simulink model "RRmanipulatorsim_"  (R2020a)
settings: Solver=VariableStepAuto  StartTime=0.0  StopTime=7  RelTol=1e-3
values from neighbouring files (symbols this model uses):
  ike = ke^(-1)    (= 1e-06)    [RRmanipulator.m]    (also in RRmanipulator_.m)
  Ke = [1e6 0; 0 0]    [RRmanipulator.m]    (also in RRmanipulator_.m)
  ke = 1e6    (= 1000000)    [RRmanipulator.m]    (also in RRmanipulator_.m)
  Kp = [g1 0; 0 g2]    [RRmanipulator.m]    (also in RRmanipulator_.m)
  Kpf = [g1f 0; 0 g2f]    [RRmanipulator.m]    (also in RRmanipulator_.m)
  Kpf_ = g1f    (= 500000)    [RRmanipulator.m]    (also in RRmanipulator_.m)
  Kv = [2*sqrt(g1) 0; 0 2*sqrt(g2)]    [RRmanipulator.m]    (also in RRmanipulator_.m)
  Kvf = [2*sqrt(g1f) 0; 0 2*sqrt(g2f)]    [RRmanipulator.m]    (also in RRmanipulator_.m)
  R = [cos(-pi/4) -sin(-pi/4) ... (first row only)    [RRmanipulator.m]    (also in RRmanipulator_.m)
  RT = R'    [RRmanipulator.m]    (also in RRmanipulator_.m)
  S = [0 0; 0 1]    [RRmanipulator.m]    (also in RRmanipulator_.m)
  S_ = [1 0; 0 0]    [RRmanipulator.m]    (also in RRmanipulator_.m)
libraries: roblocks x52, simulink x18
(part 2 of 3)

== matlab function RRmanipulatorsim_/MATLAB Function35 ==
  data: q input; taux output; qd input
function taux = Vx_Fx(q, qd)
    L = [1 1]; %Links long.
    m = [1 1]; %Links weight.
    
    M = [L(2)*m(2)*(L(2)+cos(q(2))*L(1))+m(1)*L(1)^2+L(1)*m(2)*(L(1)+cos(q(2))*L(2)) L(2)^2*m(2)+L(1)*m(2)*L(2)*cos(q(2));
        L(2)*m(2)*(L(2)+cos(q(2))*L(1)) L(2)^2*m(2)];
    V = [-2*m(2)*L(1)*L(2)*sin(q(2))*prod(qd)-m(2)*L(1)*L(2)*sin(q(2))*qd(2)^2;
        m(2)*L(1)*L(2)*sin(q(2))*qd(1)^2];
    G = [0;
        0];
    F = [sign(qd(1));
        sign(qd(2))];
    J = [-sin(sum(q))*L(2)-sin(q(1))*L(1) -sin(sum(q))*L(2);
        cos(sum(q))*L(2)+cos(q(1))*L(1) cos(sum(q))*L(2)];
    iJ = J^(-1);
    iJT = (J')^(-1);
    dJ = [-(sum(qd))*cos(sum(q))*L(2)-qd(1)*cos(q(1))*L(1) -(sum(qd))*cos(sum(q))*L(2);
        -(sum(qd))*sin(sum(q))*L(2)-qd(1)*sin(q(1))*L(1) -(sum(qd))*sin(sum(q))*L(2)];
    
    %dJqd = [dJ(1,1)*qd(1)+dJ(1,2)*qd(2); dJ(2,1)*qd(1)+dJ(2,2)*qd(2)];
    Vx = M*iJ*dJ;
    Vx = V - [Vx(1,1)*qd(1)+Vx(1,2)*qd(2); Vx(2,1)*qd(1)+Vx(2,2)*qd(2)];
    Vx = [iJT(1,1)*Vx(1)+iJT(1,2)*Vx(2); iJT(2,1)*Vx(1)+iJT(2,2)*Vx(2)];
    Gx = [iJT(1,1)*G(1)+iJT(1,2)*G(2); iJT(2,1)*G(1)+iJT(2,2)*G(2)];
    Fx = [iJT(1,1)*F(1)+iJT(1,2)*F(2); iJT(2,1)*F(1)+iJT(2,2)*F(2)];
taux = Vx + Gx + Fx;

% function taux = Vx_Fx(q, qd)
%     C = RRbot.coriolis(q', qd');
%     V = [C(1,1)*qd(1)+C(1,2)*qd(2); C(2,1)*qd(1)+C(2,2)*qd(2)]; %V = Cqd
%     F = -RRbot.friction(qd')';
%     J = RRbot.jacob0(q');
%     J = J(1:N,1:N);
%     iJ = J^(-1);
%     iJT = J.'^(-1);
%     dJ = [-(sum(qd))*cos(sum(q))*LT-qd(1)*cos(q(1))*L1 -(sum(qd))*cos(sum(q))*LT;
%         -(sum(qd))*sin(sum(q))*LT-qd(1)*sin(q(1))*L1 -(sum(qd))*sin(sum(q))*LT];
%     dJqd = [dJ(1,1)*qd(1)+dJ(1,2)*qd(2); dJ(2,1)*qd(1)+dJ(2,2)*qd(2)];
%     
%     Vx = M*iJ;
%     Vx = V - [Vx(1,1)*dJqd(1)+Vx(1,2)*dJqd(2); Vx(2,1)*dJqd(1)+Vx(2,2)*dJqd(2)];
%     Vx = [iJT(1,1)*Vx(1)+iJT(1,2)*Vx(2); iJT(2,1)*Vx(1)+iJT(2,2)*Vx(2)];
%     Fx = [iJT(1,1)*F(1)+iJT(1,2)*F(2); iJT(2,1)*F(1)+iJT(2,2)*F(2)];
% taux = Vx + Fx;

== matlab function RRmanipulatorsim_/MATLAB Function36 ==
  data: q input; x output
function x = kine(q)
    L = [1 1]; %Links long.

x = [cos(sum(q))*L(2)+cos(q(1))*L(1); sin(sum(q))*L(2)+sin(q(1))*L(1)];

== matlab function RRmanipulatorsim_/MATLAB Function37 ==
  data: q input; xd output; qd input
function xd = J(q, qd)
    L = [1 1]; %Links long.

    J = [-sin(sum(q))*L(2)-sin(q(1))*L(1) -sin(sum(q))*L(2);
        cos(sum(q))*L(2)+cos(q(1))*L(1) cos(sum(q))*L(2)];
xd = [J(1,1)*qd(1)+J(1,2)*qd(2); J(2,1)*qd(1)+J(2,2)*qd(2)];

== matlab function RRmanipulatorsim_/MATLAB Function38 ==
  data: q input; tau output; f input
function tau = JT(q, f)    
    L = [1 1]; %Links long.

    J = [-sin(sum(q))*L(2)-sin(q(1))*L(1) -sin(sum(q))*L(2);
        cos(sum(q))*L(2)+cos(q(1))*L(1) cos(sum(q))*L(2)];
    JT = J';
tau = [JT(1,1)*f(1)+JT(1,2)*f(2); JT(2,1)*f(1)+JT(2,2)*f(2)];

% function tau = JT(q, taux)
%     J = RRbot.jacob0(q');
%     JT = J(1:N,1:N)';
% tau = [JT(1,1)*taux(1)+JT(1,2)*taux(2); JT(2,1)*taux(1)+JT(2,2)*taux(2)];

== matlab function RRmanipulatorsim_/MATLAB Function39 ==
  data: q input; taux output; xdd input
function taux = Mx(q, xdd)
    L = [1 1]; %Links long.
    m = [1 1]; %Links weight.
    
    M = [L(2)*m(2)*(L(2)+cos(q(2))*L(1))+m(1)*L(1)^2+L(1)*m(2)*(L(1)+cos(q(2))*L(2)) L(2)^2*m(2)+L(1)*m(2)*L(2)*cos(q(2));
        L(2)*m(2)*(L(2)+cos(q(2))*L(1)) L(2)^2*m(2)];
    J = [-sin(sum(q))*L(2)-sin(q(1))*L(1) -sin(sum(q))*L(2);
        cos(sum(q))*L(2)+cos(q(1))*L(1) cos(sum(q))*L(2)];
    iJ = J^(-1);
    iJT = (J.')^(-1);
    
    Mx = iJT*M*iJ;
taux = [Mx(1,1)*xdd(1)+Mx(1,2)*xdd(2); Mx(2,1)*xdd(1)+Mx(2,2)*xdd(2)];

% function taux = Mx(q, xdd)
%     M = RRbot.inertia(q');
%     J = RRbot.jacob0(q');
%     J = J(1:N,1:N);
%     iJ = J^(-1);
%     iJT = J.'^(-1);
%     
%     Mx = iJT*M.*iJ;
% taux = [Mx(1,1)*xdd(1)+Mx(1,2)*xdd(2); Mx(2,1)*xdd(1)+Mx(2,2)*xdd(2)];

== matlab function RRmanipulatorsim_/MATLAB Function40 ==
  data: q input; taux output; qd input
function taux = Vx_Fx(q, qd)
    L = [1 1]; %Links long.
    m = [1 1]; %Links weight.
    
    M = [L(2)*m(2)*(L(2)+cos(q(2))*L(1))+m(1)*L(1)^2+L(1)*m(2)*(L(1)+cos(q(2))*L(2)) L(2)^2*m(2)+L(1)*m(2)*L(2)*cos(q(2));
        L(2)*m(2)*(L(2)+cos(q(2))*L(1)) L(2)^2*m(2)];
    V = [-2*m(2)*L(1)*L(2)*sin(q(2))*prod(qd)-m(2)*L(1)*L(2)*sin(q(2))*qd(2)^2;
        m(2)*L(1)*L(2)*sin(q(2))*qd(1)^2];
    G = [0;
        0];
    F = [sign(qd(1));
        sign(qd(2))];
    J = [-sin(sum(q))*L(2)-sin(q(1))*L(1) -sin(sum(q))*L(2);
        cos(sum(q))*L(2)+cos(q(1))*L(1) cos(sum(q))*L(2)];
    iJ = J^(-1);
    iJT = (J')^(-1);
    dJ = [-(sum(qd))*cos(sum(q))*L(2)-qd(1)*cos(q(1))*L(1) -(sum(qd))*cos(sum(q))*L(2);
        -(sum(qd))*sin(sum(q))*L(2)-qd(1)*sin(q(1))*L(1) -(sum(qd))*sin(sum(q))*L(2)];
    
    %dJqd = [dJ(1,1)*qd(1)+dJ(1,2)*qd(2); dJ(2,1)*qd(1)+dJ(2,2)*qd(2)];
    Vx = M*iJ*dJ;
    Vx = V - [Vx(1,1)*qd(1)+Vx(1,2)*qd(2); Vx(2,1)*qd(1)+Vx(2,2)*qd(2)];
    Vx = [iJT(1,1)*Vx(1)+iJT(1,2)*Vx(2); iJT(2,1)*Vx(1)+iJT(2,2)*Vx(2)];
    Gx = [iJT(1,1)*G(1)+iJT(1,2)*G(2); iJT(2,1)*G(1)+iJT(2,2)*G(2)];
    Fx = [iJT(1,1)*F(1)+iJT(1,2)*F(2); iJT(2,1)*F(1)+iJT(2,2)*F(2)];
taux = Vx + Gx + Fx;

% function taux = Vx_Fx(q, qd)
%     C = RRbot.coriolis(q', qd');
%     V = [C(1,1)*qd(1)+C(1,2)*qd(2); C(2,1)*qd(1)+C(2,2)*qd(2)]; %V = Cqd
%     F = -RRbot.friction(qd')';
%     J = RRbot.jacob0(q');
%     J = J(1:N,1:N);
%     iJ = J^(-1);
%     iJT = J.'^(-1);
%     dJ = [-(sum(qd))*cos(sum(q))*LT-qd(1)*cos(q(1))*L1 -(sum(qd))*cos(sum(q))*LT;
%         -(sum(qd))*sin(sum(q))*LT-qd(1)*sin(q(1))*L1 -(sum(qd))*sin(sum(q))*LT];
%     dJqd = [dJ(1,1)*qd(1)+dJ(1,2)*qd(2); dJ(2,1)*qd(1)+dJ(2,2)*qd(2)];
%     
%     Vx = M*iJ;
%     Vx = V - [Vx(1,1)*dJqd(1)+Vx(1,2)*dJqd(2); Vx(2,1)*dJqd(1)+Vx(2,2)*dJqd(2)];
%     Vx = [iJT(1,1)*Vx(1)+iJT(1,2)*Vx(2); iJT(2,1)*Vx(1)+iJT(2,2)*Vx(2)];
%     Fx = [iJT(1,1)*F(1)+iJT(1,2)*F(2); iJT(2,1)*F(1)+iJT(2,2)*F(2)];
% taux = Vx + Fx;

== matlab function RRmanipulatorsim_/MATLAB Function41 ==
  data: q input; x output
function x = kine(q)
    L = [1 1]; %Links long.

x = [cos(sum(q))*L(2)+cos(q(1))*L(1); sin(sum(q))*L(2)+sin(q(1))*L(1)];

== matlab function RRmanipulatorsim_/MATLAB Function42 ==
  data: q input; xd output; qd input
function xd = J(q, qd)
    L = [1 1]; %Links long.

    J = [-sin(sum(q))*L(2)-sin(q(1))*L(1) -sin(sum(q))*L(2);
        cos(sum(q))*L(2)+cos(q(1))*L(1) cos(sum(q))*L(2)];
xd = [J(1,1)*qd(1)+J(1,2)*qd(2); J(2,1)*qd(1)+J(2,2)*qd(2)];

== matlab function RRmanipulatorsim_/MATLAB Function3 ==
  data: q input; taux output; qd input
function taux = Vx_Fx(q, qd)
    L = [1 1]; %Links long.
    m = [1 1]; %Links weight.
    
    M = [L(2)*m(2)*(L(2)+cos(q(2))*L(1))+m(1)*L(1)^2+L(1)*m(2)*(L(1)+cos(q(2))*L(2)) L(2)^2*m(2)+L(1)*m(2)*L(2)*cos(q(2));
        L(2)*m(2)*(L(2)+cos(q(2))*L(1)) L(2)^2*m(2)];
    V = [-2*m(2)*L(1)*L(2)*sin(q(2))*prod(qd)-m(2)*L(1)*L(2)*sin(q(2))*qd(2)^2;
        m(2)*L(1)*L(2)*sin(q(2))*qd(1)^2];
    G = [0;
        0];
    F = [sign(qd(1));
        sign(qd(2))];
    J = [-sin(sum(q))*L(2)-sin(q(1))*L(1) -sin(sum(q))*L(2);
        cos(sum(q))*L(2)+cos(q(1))*L(1) cos(sum(q))*L(2)];
    iJ = J^(-1);
    iJT = (J')^(-1);
    dJ = [-(sum(qd))*cos(sum(q))*L(2)-qd(1)*cos(q(1))*L(1) -(sum(qd))*cos(sum(q))*L(2);
        -(sum(qd))*sin(sum(q))*L(2)-qd(1)*sin(q(1))*L(1) -(sum(qd))*sin(sum(q))*L(2)];
    
    %dJqd = [dJ(1,1)*qd(1)+dJ(1,2)*qd(2); dJ(2,1)*qd(1)+dJ(2,2)*qd(2)];
    Vx = M*iJ*dJ;
    Vx = V - [Vx(1,1)*qd(1)+Vx(1,2)*qd(2); Vx(2,1)*qd(1)+Vx(2,2)*qd(2)];
    Vx = [iJT(1,1)*Vx(1)+iJT(1,2)*Vx(2); iJT(2,1)*Vx(1)+iJT(2,2)*Vx(2)];
    Gx = [iJT(1,1)*G(1)+iJT(1,2)*G(2); iJT(2,1)*G(1)+iJT(2,2)*G(2)];
    Fx = [iJT(1,1)*F(1)+iJT(1,2)*F(2); iJT(2,1)*F(1)+iJT(2,2)*F(2)];
taux = Vx + Gx + Fx;

% function taux = Vx_Fx(q, qd)
%     C = RRbot.coriolis(q', qd');
%     V = [C(1,1)*qd(1)+C(1,2)*qd(2); C(2,1)*qd(1)+C(2,2)*qd(2)]; %V = Cqd
%     F = -RRbot.friction(qd')';
%     J = RRbot.jacob0(q');
%     J = J(1:N,1:N);
%     iJ = J^(-1);
%     iJT = J.'^(-1);
%     dJ = [-(sum(qd))*cos(sum(q))*LT-qd(1)*cos(q(1))*L1 -(sum(qd))*cos(sum(q))*LT;
%         -(sum(qd))*sin(sum(q))*LT-qd(1)*sin(q(1))*L1 -(sum(qd))*sin(sum(q))*LT];
%     dJqd = [dJ(1,1)*qd(1)+dJ(1,2)*qd(2); dJ(2,1)*qd(1)+dJ(2,2)*qd(2)];
%     
%     Vx = M*iJ;
%     Vx = V - [Vx(1,1)*dJqd(1)+Vx(1,2)*dJqd(2); Vx(2,1)*dJqd(1)+Vx(2,2)*dJqd(2)];
%     Vx = [iJT(1,1)*Vx(1)+iJT(1,2)*Vx(2); iJT(2,1)*Vx(1)+iJT(2,2)*Vx(2)];
%     Fx = [iJT(1,1)*F(1)+iJT(1,2)*F(2); iJT(2,1)*F(1)+iJT(2,2)*F(2)];
% taux = Vx + Fx;

== matlab function RRmanipulatorsim_/MATLAB Function43 ==
  data: q input; tau output; f input
function tau = JT(q, f)    
    L = [1 1]; %Links long.

    J = [-sin(sum(q))*L(2)-sin(q(1))*L(1) -sin(sum(q))*L(2);
        cos(sum(q))*L(2)+cos(q(1))*L(1) cos(sum(q))*L(2)];
    JT = J';
tau = [JT(1,1)*f(1)+JT(1,2)*f(2); JT(2,1)*f(1)+JT(2,2)*f(2)];

% function tau = JT(q, taux)
%     J = RRbot.jacob0(q');
%     JT = J(1:N,1:N)';
% tau = [JT(1,1)*taux(1)+JT(1,2)*taux(2); JT(2,1)*taux(1)+JT(2,2)*taux(2)];

== matlab function RRmanipulatorsim_/MATLAB Function44 ==
  data: q input; taux output; xdd input
function taux = Mx(q, xdd)
    L = [1 1]; %Links long.
    m = [1 1]; %Links weight.
    
    M = [L(2)*m(2)*(L(2)+cos(q(2))*L(1))+m(1)*L(1)^2+L(1)*m(2)*(L(1)+cos(q(2))*L(2)) L(2)^2*m(2)+L(1)*m(2)*L(2)*cos(q(2));
        L(2)*m(2)*(L(2)+cos(q(2))*L(1)) L(2)^2*m(2)];
    J = [-sin(sum(q))*L(2)-sin(q(1))*L(1) -sin(sum(q))*L(2);
        cos(sum(q))*L(2)+cos(q(1))*L(1) cos(sum(q))*L(2)];
    iJ = J^(-1);
    iJT = (J.')^(-1);
    
    Mx = iJT*M*iJ;
taux = [Mx(1,1)*xdd(1)+Mx(1,2)*xdd(2); Mx(2,1)*xdd(1)+Mx(2,2)*xdd(2)];

% function taux = Mx(q, xdd)
%     M = RRbot.inertia(q');
%     J = RRbot.jacob0(q');
%     J = J(1:N,1:N);
%     iJ = J^(-1);
%     iJT = J.'^(-1);
%     
%     Mx = iJT*M.*iJ;
% taux = [Mx(1,1)*xdd(1)+Mx(1,2)*xdd(2); Mx(2,1)*xdd(1)+Mx(2,2)*xdd(2)];

== matlab function RRmanipulatorsim_/MATLAB Function45 ==
  data: q input; taux output; qd input
function taux = Vx_Fx(q, qd)
    L = [1 1]; %Links long.
    m = [1 1]; %Links weight.
    
    M = [L(2)*m(2)*(L(2)+cos(q(2))*L(1))+m(1)*L(1)^2+L(1)*m(2)*(L(1)+cos(q(2))*L(2)) L(2)^2*m(2)+L(1)*m(2)*L(2)*cos(q(2));
        L(2)*m(2)*(L(2)+cos(q(2))*L(1)) L(2)^2*m(2)];
    V = [-2*m(2)*L(1)*L(2)*sin(q(2))*prod(qd)-m(2)*L(1)*L(2)*sin(q(2))*qd(2)^2;
        m(2)*L(1)*L(2)*sin(q(2))*qd(1)^2];
    G = [0;
        0];
    F = [sign(qd(1));
        sign(qd(2))];
    J = [-sin(sum(q))*L(2)-sin(q(1))*L(1) -sin(sum(q))*L(2);
        cos(sum(q))*L(2)+cos(q(1))*L(1) cos(sum(q))*L(2)];
    iJ = J^(-1);
    iJT = (J')^(-1);
    dJ = [-(sum(qd))*cos(sum(q))*L(2)-qd(1)*cos(q(1))*L(1) -(sum(qd))*cos(sum(q))*L(2);
        -(sum(qd))*sin(sum(q))*L(2)-qd(1)*sin(q(1))*L(1) -(sum(qd))*sin(sum(q))*L(2)];
    
    %dJqd = [dJ(1,1)*qd(1)+dJ(1,2)*qd(2); dJ(2,1)*qd(1)+dJ(2,2)*qd(2)];
    Vx = M*iJ*dJ;
    Vx = V - [Vx(1,1)*qd(1)+Vx(1,2)*qd(2); Vx(2,1)*qd(1)+Vx(2,2)*qd(2)];
    Vx = [iJT(1,1)*Vx(1)+iJT(1,2)*Vx(2); iJT(2,1)*Vx(1)+iJT(2,2)*Vx(2)];
    Gx = [iJT(1,1)*G(1)+iJT(1,2)*G(2); iJT(2,1)*G(1)+iJT(2,2)*G(2)];
    Fx = [iJT(1,1)*F(1)+iJT(1,2)*F(2); iJT(2,1)*F(1)+iJT(2,2)*F(2)];
taux = Vx + Gx + Fx;

% function taux = Vx_Fx(q, qd)
%     C = RRbot.coriolis(q', qd');
%     V = [C(1,1)*qd(1)+C(1,2)*qd(2); C(2,1)*qd(1)+C(2,2)*qd(2)]; %V = Cqd
%     F = -RRbot.friction(qd')';
%     J = RRbot.jacob0(q');
%     J = J(1:N,1:N);
%     iJ = J^(-1);
%     iJT = J.'^(-1);
%     dJ = [-(sum(qd))*cos(sum(q))*LT-qd(1)*cos(q(1))*L1 -(sum(qd))*cos(sum(q))*LT;
%         -(sum(qd))*sin(sum(q))*LT-qd(1)*sin(q(1))*L1 -(sum(qd))*sin(sum(q))*LT];
%     dJqd = [dJ(1,1)*qd(1)+dJ(1,2)*qd(2); dJ(2,1)*qd(1)+dJ(2,2)*qd(2)];
%     
%     Vx = M*iJ;
%     Vx = V - [Vx(1,1)*dJqd(1)+Vx(1,2)*dJqd(2); Vx(2,1)*dJqd(1)+Vx(2,2)*dJqd(2)];
%     Vx = [iJT(1,1)*Vx(1)+iJT(1,2)*Vx(2); iJT(2,1)*Vx(1)+iJT(2,2)*Vx(2)];
%     Fx = [iJT(1,1)*F(1)+iJT(1,2)*F(2); iJT(2,1)*F(1)+iJT(2,2)*F(2)];
% taux = Vx + Fx;

== matlab function RRmanipulatorsim_/MATLAB Function46 ==
  data: q input; x output
function x = kine(q)
    L = [1 1]; %Links long.

x = [cos(sum(q))*L(2)+cos(q(1))*L(1); sin(sum(q))*L(2)+sin(q(1))*L(1)];

== matlab function RRmanipulatorsim_/MATLAB Function47 ==
  data: q input; xd output; qd input
function xd = J(q, qd)
    L = [1 1]; %Links long.

    J = [-sin(sum(q))*L(2)-sin(q(1))*L(1) -sin(sum(q))*L(2);
        cos(sum(q))*L(2)+cos(q(1))*L(1) cos(sum(q))*L(2)];
xd = [J(1,1)*qd(1)+J(1,2)*qd(2); J(2,1)*qd(1)+J(2,2)*qd(2)];

== matlab function RRmanipulatorsim_/MATLAB Function48 ==
  data: q input; tau output; f input
function tau = JT(q, f)    
    L = [1 1]; %Links long.

    J = [-sin(sum(q))*L(2)-sin(q(1))*L(1) -sin(sum(q))*L(2);
        cos(sum(q))*L(2)+cos(q(1))*L(1) cos(sum(q))*L(2)];
    JT = J';
tau = [JT(1,1)*f(1)+JT(1,2)*f(2); JT(2,1)*f(1)+JT(2,2)*f(2)];

% function tau = JT(q, taux)
%     J = RRbot.jacob0(q');
%     JT = J(1:N,1:N)';
% tau = [JT(1,1)*taux(1)+JT(1,2)*taux(2); JT(2,1)*taux(1)+JT(2,2)*taux(2)];

== matlab function RRmanipulatorsim_/MATLAB Function49 ==
  data: x input; f output
function f = Ke(x)
    Ke = 1e6;

f = Ke*x;

== matlab function RRmanipulatorsim_/MATLAB Function50 ==
  data: f input; x output
function x = iKe(f)
    Ke = 1e6;
    
    iKe = Ke^(-1);
x = f*iKe;

== matlab function RRmanipulatorsim_/MATLAB Function51 ==
  data: x input; x_ output
function x_ = R(x)
    R = [cos(-pi/4) -sin(-pi/4);
        sin(-pi/4) cos(-pi/4)];
x_ = [R(1,1)*x(1)+R(1,2)*x(2); R(2,1)*x(1)+R(2,2)*x(2)];

== matlab function RRmanipulatorsim_/MATLAB Function52 ==
  data: x input; x_ output
function x_ = R(x)
    R = [cos(-pi/4) -sin(-pi/4);
        sin(-pi/4) cos(-pi/4)];
x_ = [R(1,1)*x(1)+R(1,2)*x(2); R(2,1)*x(1)+R(2,2)*x(2)];

== matlab function RRmanipulatorsim_/MATLAB Function4 ==
  data: q input; tau output; qdd input
function tau = M(q, qdd)
    L = [1 1]; %Links long.
    m = [1 1]; %Links weight.

    M = [L(2)*m(2)*(L(2)+cos(q(2))*L(1))+m(1)*L(1)^2+L(1)*m(2)*(L(1)+cos(q(2))*L(2)) L(2)^2*m(2)+L(1)*m(2)*L(2)*cos(q(2));
    L(2)*m(2)*(L(2)+cos(q(2))*L(1)) L(2)^2*m(2)];
    
tau = [M(1,1)*qdd(1)+M(1,2)*qdd(2); M(2,1)*qdd(1)+M(2,2)*qdd(2)];

== matlab function RRmanipulatorsim_/MATLAB Function53 ==
  data: x_ input; x output
function x = RT(x_)
    R = [cos(-pi/4) -sin(-pi/4);
        sin(-pi/4) cos(-pi/4)];
    
    RT = R';
x = [RT(1,1)*x_(1)+RT(1,2)*x_(2); RT(2,1)*x_(1)+RT(2,2)*x_(2)];

== matlab function RRmanipulatorsim_/MATLAB Function54 ==
  data: q input; taux output; xdd input
function taux = Mx(q, xdd)
    L = [1 1]; %Links long.
    m = [1 1]; %Links weight.
    
    M = [L(2)*m(2)*(L(2)+cos(q(2))*L(1))+m(1)*L(1)^2+L(1)*m(2)*(L(1)+cos(q(2))*L(2)) L(2)^2*m(2)+L(1)*m(2)*L(2)*cos(q(2));
        L(2)*m(2)*(L(2)+cos(q(2))*L(1)) L(2)^2*m(2)];
    J = [-sin(sum(q))*L(2)-sin(q(1))*L(1) -sin(sum(q))*L(2);
        cos(sum(q))*L(2)+cos(q(1))*L(1) cos(sum(q))*L(2)];
    iJ = J^(-1);
    iJT = (J.')^(-1);
    
    Mx = iJT*M*iJ;
taux = [Mx(1,1)*xdd(1)+Mx(1,2)*xdd(2); Mx(2,1)*xdd(1)+Mx(2,2)*xdd(2)];

% function taux = Mx(q, xdd)
%     M = RRbot.inertia(q');
%     J = RRbot.jacob0(q');
%     J = J(1:N,1:N);
%     iJ = J^(-1);
%     iJT = J.'^(-1);
%     
%     Mx = iJT*M.*iJ;
% taux = [Mx(1,1)*xdd(1)+Mx(1,2)*xdd(2); Mx(2,1)*xdd(1)+Mx(2,2)*xdd(2)];

== matlab function RRmanipulatorsim_/MATLAB Function55 ==
  data: q input; taux output; qd input
function taux = Vx_Fx(q, qd)
    L = [1 1]; %Links long.
    m = [1 1]; %Links weight.
    
    M = [L(2)*m(2)*(L(2)+cos(q(2))*L(1))+m(1)*L(1)^2+L(1)*m(2)*(L(1)+cos(q(2))*L(2)) L(2)^2*m(2)+L(1)*m(2)*L(2)*cos(q(2));
        L(2)*m(2)*(L(2)+cos(q(2))*L(1)) L(2)^2*m(2)];
    V = [-2*m(2)*L(1)*L(2)*sin(q(2))*prod(qd)-m(2)*L(1)*L(2)*sin(q(2))*qd(2)^2;
        m(2)*L(1)*L(2)*sin(q(2))*qd(1)^2];
    G = [0;
        0];
    F = [sign(qd(1));
        sign(qd(2))];
    J = [-sin(sum(q))*L(2)-sin(q(1))*L(1) -sin(sum(q))*L(2);
        cos(sum(q))*L(2)+cos(q(1))*L(1) cos(sum(q))*L(2)];
    iJ = J^(-1);
    iJT = (J')^(-1);
    dJ = [-(sum(qd))*cos(sum(q))*L(2)-qd(1)*cos(q(1))*L(1) -(sum(qd))*cos(sum(q))*L(2);
        -(sum(qd))*sin(sum(q))*L(2)-qd(1)*sin(q(1))*L(1) -(sum(qd))*sin(sum(q))*L(2)];
    
    %dJqd = [dJ(1,1)*qd(1)+dJ(1,2)*qd(2); dJ(2,1)*qd(1)+dJ(2,2)*qd(2)];
    Vx = M*iJ*dJ;
    Vx = V - [Vx(1,1)*qd(1)+Vx(1,2)*qd(2); Vx(2,1)*qd(1)+Vx(2,2)*qd(2)];
    Vx = [iJT(1,1)*Vx(1)+iJT(1,2)*Vx(2); iJT(2,1)*Vx(1)+iJT(2,2)*Vx(2)];
    Gx = [iJT(1,1)*G(1)+iJT(1,2)*G(2); iJT(2,1)*G(1)+iJT(2,2)*G(2)];
    Fx = [iJT(1,1)*F(1)+iJT(1,2)*F(2); iJT(2,1)*F(1)+iJT(2,2)*F(2)];
taux = Vx + Gx + Fx;

% function taux = Vx_Fx(q, qd)
%     C = RRbot.coriolis(q', qd');
%     V = [C(1,1)*qd(1)+C(1,2)*qd(2); C(2,1)*qd(1)+C(2,2)*qd(2)]; %V = Cqd
%     F = -RRbot.friction(qd')';
%     J = RRbot.jacob0(q');
%     J = J(1:N,1:N);
%     iJ = J^(-1);
%     iJT = J.'^(-1);
%     dJ = [-(sum(qd))*cos(sum(q))*LT-qd(1)*cos(q(1))*L1 -(sum(qd))*cos(sum(q))*LT;
%         -(sum(qd))*sin(sum(q))*LT-qd(1)*sin(q(1))*L1 -(sum(qd))*sin(sum(q))*LT];
%     dJqd = [dJ(1,1)*qd(1)+dJ(1,2)*qd(2); dJ(2,1)*qd(1)+dJ(2,2)*qd(2)];
%     
%     Vx = M*iJ;
%     Vx = V - [Vx(1,1)*dJqd(1)+Vx(1,2)*dJqd(2); Vx(2,1)*dJqd(1)+Vx(2,2)*dJqd(2)];
%     Vx = [iJT(1,1)*Vx(1)+iJT(1,2)*Vx(2); iJT(2,1)*Vx(1)+iJT(2,2)*Vx(2)];
%     Fx = [iJT(1,1)*F(1)+iJT(1,2)*F(2); iJT(2,1)*F(1)+iJT(2,2)*F(2)];
% taux = Vx + Fx;

== matlab function RRmanipulatorsim_/MATLAB Function56 ==
  data: q input; x output
function x = kine(q)
    L = [1 1]; %Links long.

x = [cos(sum(q))*L(2)+cos(q(1))*L(1); sin(sum(q))*L(2)+sin(q(1))*L(1)];

== matlab function RRmanipulatorsim_/MATLAB Function57 ==
  data: q input; xd output; qd input
function xd = J(q, qd)
    L = [1 1]; %Links long.

    J = [-sin(sum(q))*L(2)-sin(q(1))*L(1) -sin(sum(q))*L(2);
        cos(sum(q))*L(2)+cos(q(1))*L(1) cos(sum(q))*L(2)];
xd = [J(1,1)*qd(1)+J(1,2)*qd(2); J(2,1)*qd(1)+J(2,2)*qd(2)];

== matlab function RRmanipulatorsim_/MATLAB Function58 ==
  data: q input; tau output; f input
function tau = JT(q, f)    
    L = [1 1]; %Links long.

    J = [-sin(sum(q))*L(2)-sin(q(1))*L(1) -sin(sum(q))*L(2);
        cos(sum(q))*L(2)+cos(q(1))*L(1) cos(sum(q))*L(2)];
    JT = J';
tau = [JT(1,1)*f(1)+JT(1,2)*f(2); JT(2,1)*f(1)+JT(2,2)*f(2)];

% function tau = JT(q, taux)
%     J = RRbot.jacob0(q');
%     JT = J(1:N,1:N)';
% tau = [JT(1,1)*taux(1)+JT(1,2)*taux(2); JT(2,1)*taux(1)+JT(2,2)*taux(2)];

== matlab function RRmanipulatorsim_/MATLAB Function59 ==
  data: q input; taux output; xdd input
function taux = Mx(q, xdd)
    L = [1 1]; %Links long.
    m = [1 1]; %Links weight.
    
    M = [L(2)*m(2)*(L(2)+cos(q(2))*L(1))+m(1)*L(1)^2+L(1)*m(2)*(L(1)+cos(q(2))*L(2)) L(2)^2*m(2)+L(1)*m(2)*L(2)*cos(q(2));
        L(2)*m(2)*(L(2)+cos(q(2))*L(1)) L(2)^2*m(2)];
    J = [-sin(sum(q))*L(2)-sin(q(1))*L(1) -sin(sum(q))*L(2);
        cos(sum(q))*L(2)+cos(q(1))*L(1) cos(sum(q))*L(2)];
    iJ = J^(-1);
    iJT = (J.')^(-1);
    
    Mx = iJT*M*iJ;
taux = [Mx(1,1)*xdd(1)+Mx(1,2)*xdd(2); Mx(2,1)*xdd(1)+Mx(2,2)*xdd(2)];

% function taux = Mx(q, xdd)
%     M = RRbot.inertia(q');
%     J = RRbot.jacob0(q');
%     J = J(1:N,1:N);
%     iJ = J^(-1);
%     iJT = J.'^(-1);
%     
%     Mx = iJT*M.*iJ;
% taux = [Mx(1,1)*xdd(1)+Mx(1,2)*xdd(2); Mx(2,1)*xdd(1)+Mx(2,2)*xdd(2)];

== matlab function RRmanipulatorsim_/MATLAB Function60 ==
  data: q input; taux output; qd input
function taux = Vx_Fx(q, qd)
    L = [1 1]; %Links long.
    m = [1 1]; %Links weight.
    
    M = [L(2)*m(2)*(L(2)+cos(q(2))*L(1))+m(1)*L(1)^2+L(1)*m(2)*(L(1)+cos(q(2))*L(2)) L(2)^2*m(2)+L(1)*m(2)*L(2)*cos(q(2));
        L(2)*m(2)*(L(2)+cos(q(2))*L(1)) L(2)^2*m(2)];
    V = [-2*m(2)*L(1)*L(2)*sin(q(2))*prod(qd)-m(2)*L(1)*L(2)*sin(q(2))*qd(2)^2;
        m(2)*L(1)*L(2)*sin(q(2))*qd(1)^2];
    G = [0;
        0];
    F = [sign(qd(1));
        sign(qd(2))];
    J = [-sin(sum(q))*L(2)-sin(q(1))*L(1) -sin(sum(q))*L(2);
        cos(sum(q))*L(2)+cos(q(1))*L(1) cos(sum(q))*L(2)];
    iJ = J^(-1);
    iJT = (J')^(-1);
    dJ = [-(sum(qd))*cos(sum(q))*L(2)-qd(1)*cos(q(1))*L(1) -(sum(qd))*cos(sum(q))*L(2);
        -(sum(qd))*sin(sum(q))*L(2)-qd(1)*sin(q(1))*L(1) -(sum(qd))*sin(sum(q))*L(2)];
    
    %dJqd = [dJ(1,1)*qd(1)+dJ(1,2)*qd(2); dJ(2,1)*qd(1)+dJ(2,2)*qd(2)];
    Vx = M*iJ*dJ;
    Vx = V - [Vx(1,1)*qd(1)+Vx(1,2)*qd(2); Vx(2,1)*qd(1)+Vx(2,2)*qd(2)];
    Vx = [iJT(1,1)*Vx(1)+iJT(1,2)*Vx(2); iJT(2,1)*Vx(1)+iJT(2,2)*Vx(2)];
    Gx = [iJT(1,1)*G(1)+iJT(1,2)*G(2); iJT(2,1)*G(1)+iJT(2,2)*G(2)];
    Fx = [iJT(1,1)*F(1)+iJT(1,2)*F(2); iJT(2,1)*F(1)+iJT(2,2)*F(2)];
taux = Vx + Gx + Fx;

% function taux = Vx_Fx(q, qd)
%     C = RRbot.coriolis(q', qd');
%     V = [C(1,1)*qd(1)+C(1,2)*qd(2); C(2,1)*qd(1)+C(2,2)*qd(2)]; %V = Cqd
%     F = -RRbot.friction(qd')';
%     J = RRbot.jacob0(q');
%     J = J(1:N,1:N);
%     iJ = J^(-1);
%     iJT = J.'^(-1);
%     dJ = [-(sum(qd))*cos(sum(q))*LT-qd(1)*cos(q(1))*L1 -(sum(qd))*cos(sum(q))*LT;
%         -(sum(qd))*sin(sum(q))*LT-qd(1)*sin(q(1))*L1 -(sum(qd))*sin(sum(q))*LT];
%     dJqd = [dJ(1,1)*qd(1)+dJ(1,2)*qd(2); dJ(2,1)*qd(1)+dJ(2,2)*qd(2)];
%     
%     Vx = M*iJ;
%     Vx = V - [Vx(1,1)*dJqd(1)+Vx(1,2)*dJqd(2); Vx(2,1)*dJqd(1)+Vx(2,2)*dJqd(2)];
%     Vx = [iJT(1,1)*Vx(1)+iJT(1,2)*Vx(2); iJT(2,1)*Vx(1)+iJT(2,2)*Vx(2)];
%     Fx = [iJT(1,1)*F(1)+iJT(1,2)*F(2); iJT(2,1)*F(1)+iJT(2,2)*F(2)];
% taux = Vx + Fx;

== matlab function RRmanipulatorsim_/MATLAB Function61 ==
  data: q input; taux output; xdd input
function taux = Mx(q, xdd)
    L = [1 1]; %Links long.
    m = [1 1]; %Links weight.
    
    M = [L(2)*m(2)*(L(2)+cos(q(2))*L(1))+m(1)*L(1)^2+L(1)*m(2)*(L(1)+cos(q(2))*L(2)) L(2)^2*m(2)+L(1)*m(2)*L(2)*cos(q(2));
        L(2)*m(2)*(L(2)+cos(q(2))*L(1)) L(2)^2*m(2)];
    J = [-sin(sum(q))*L(2)-sin(q(1))*L(1) -sin(sum(q))*L(2);
        cos(sum(q))*L(2)+cos(q(1))*L(1) cos(sum(q))*L(2)];
    iJ = J^(-1);
    iJT = (J.')^(-1);
    
    Mx = iJT*M*iJ;
taux = [Mx(1,1)*xdd(1)+Mx(1,2)*xdd(2); Mx(2,1)*xdd(1)+Mx(2,2)*xdd(2)];

% function taux = Mx(q, xdd)
%     M = RRbot.inertia(q');
%     J = RRbot.jacob0(q');
%     J = J(1:N,1:N);
%     iJ = J^(-1);
%     iJT = J.'^(-1);
%     
%     Mx = iJT*M.*iJ;
% taux = [Mx(1,1)*xdd(1)+Mx(1,2)*xdd(2); Mx(2,1)*xdd(1)+Mx(2,2)*xdd(2)];

== matlab function RRmanipulatorsim_/MATLAB Function62 ==
  data: q input; taux output; qd input
function taux = Vx_Fx(q, qd)
    L = [1 1]; %Links long.
    m = [1 1]; %Links weight.
    
    M = [L(2)*m(2)*(L(2)+cos(q(2))*L(1))+m(1)*L(1)^2+L(1)*m(2)*(L(1)+cos(q(2))*L(2)) L(2)^2*m(2)+L(1)*m(2)*L(2)*cos(q(2));
        L(2)*m(2)*(L(2)+cos(q(2))*L(1)) L(2)^2*m(2)];
    V = [-2*m(2)*L(1)*L(2)*sin(q(2))*prod(qd)-m(2)*L(1)*L(2)*sin(q(2))*qd(2)^2;
        m(2)*L(1)*L(2)*sin(q(2))*qd(1)^2];
    G = [0;
        0];
    F = [sign(qd(1));
        sign(qd(2))];
    J = [-sin(sum(q))*L(2)-sin(q(1))*L(1) -sin(sum(q))*L(2);
        cos(sum(q))*L(2)+cos(q(1))*L(1) cos(sum(q))*L(2)];
    iJ = J^(-1);
    iJT = (J')^(-1);
    dJ = [-(sum(qd))*cos(sum(q))*L(2)-qd(1)*cos(q(1))*L(1) -(sum(qd))*cos(sum(q))*L(2);
        -(sum(qd))*sin(sum(q))*L(2)-qd(1)*sin(q(1))*L(1) -(sum(qd))*sin(sum(q))*L(2)];
    
    %dJqd = [dJ(1,1)*qd(1)+dJ(1,2)*qd(2); dJ(2,1)*qd(1)+dJ(2,2)*qd(2)];
    Vx = M*iJ*dJ;
    Vx = V - [Vx(1,1)*qd(1)+Vx(1,2)*qd(2); Vx(2,1)*qd(1)+Vx(2,2)*qd(2)];
    Vx = [iJT(1,1)*Vx(1)+iJT(1,2)*Vx(2); iJT(2,1)*Vx(1)+iJT(2,2)*Vx(2)];
    Gx = [iJT(1,1)*G(1)+iJT(1,2)*G(2); iJT(2,1)*G(1)+iJT(2,2)*G(2)];
    Fx = [iJT(1,1)*F(1)+iJT(1,2)*F(2); iJT(2,1)*F(1)+iJT(2,2)*F(2)];
taux = Vx + Gx + Fx;

% function taux = Vx_Fx(q, qd)
%     C = RRbot.coriolis(q', qd');
%     V = [C(1,1)*qd(1)+C(1,2)*qd(2); C(2,1)*qd(1)+C(2,2)*qd(2)]; %V = Cqd
%     F = -RRbot.friction(qd')';
%     J = RRbot.jacob0(q');
%     J = J(1:N,1:N);
%     iJ = J^(-1);
%     iJT = J.'^(-1);
%     dJ = [-(sum(qd))*cos(sum(q))*LT-qd(1)*cos(q(1))*L1 -(sum(qd))*cos(sum(q))*LT;
%         -(sum(qd))*sin(sum(q))*LT-qd(1)*sin(q(1))*L1 -(sum(qd))*sin(sum(q))*LT];
%     dJqd = [dJ(1,1)*qd(1)+dJ(1,2)*qd(2); dJ(2,1)*qd(1)+dJ(2,2)*qd(2)];
%     
%     Vx = M*iJ;
%     Vx = V - [Vx(1,1)*dJqd(1)+Vx(1,2)*dJqd(2); Vx(2,1)*dJqd(1)+Vx(2,2)*dJqd(2)];
%     Vx = [iJT(1,1)*Vx(1)+iJT(1,2)*Vx(2); iJT(2,1)*Vx(1)+iJT(2,2)*Vx(2)];
%     Fx = [iJT(1,1)*F(1)+iJT(1,2)*F(2); iJT(2,1)*F(1)+iJT(2,2)*F(2)];
% taux = Vx + Fx;

== matlab function RRmanipulatorsim_/MATLAB Function5 ==
  data: q input; tau output; qd input
function tau = V_F(q, qd)
    L = [1 1]; %Links long.
    m = [1 1]; %Links weight.

    V = [-2*m(2)*L(1)*L(2)*sin(q(2))*prod(qd)-m(2)*L(1)*L(2)*sin(q(2))*qd(2)^2;
        m(2)*L(1)*L(2)*sin(q(2))*qd(1)^2];

    F = [sign(qd(1));
        sign(qd(2))];
    
tau = V + F;

== matlab function RRmanipulatorsim_/MATLAB Function63 ==
  data: q input; x output
function x = kine(q)
    L = [1 1]; %Links long.

x = [cos(sum(q))*L(2)+cos(q(1))*L(1); sin(sum(q))*L(2)+sin(q(1))*L(1)];

== matlab function RRmanipulatorsim_/MATLAB Function64 ==
  data: q input; xd output; qd input
function xd = J(q, qd)
    L = [1 1]; %Links long.

    J = [-sin(sum(q))*L(2)-sin(q(1))*L(1) -sin(sum(q))*L(2);
        cos(sum(q))*L(2)+cos(q(1))*L(1) cos(sum(q))*L(2)];
xd = [J(1,1)*qd(1)+J(1,2)*qd(2); J(2,1)*qd(1)+J(2,2)*qd(2)];

== matlab function RRmanipulatorsim_/MATLAB Function65 ==
  data: q input; tau output; taux input
function tau = JT(q, taux)    
    L = [1 1]; %Links long.

    J = [-sin(sum(q))*L(2)-sin(q(1))*L(1) -sin(sum(q))*L(2);
        cos(sum(q))*L(2)+cos(q(1))*L(1) cos(sum(q))*L(2)];
    JT = J';
tau = [JT(1,1)*taux(1)+JT(1,2)*taux(2); JT(2,1)*taux(1)+JT(2,2)*taux(2)];

% function tau = JT(q, taux)
%     J = RRbot.jacob0(q');
%     JT = J(1:N,1:N)';
% tau = [JT(1,1)*taux(1)+JT(1,2)*taux(2); JT(2,1)*taux(1)+JT(2,2)*taux(2)];

== matlab function RRmanipulatorsim_/MATLAB Function66 ==
  data: x input; q output
function q = ikine(x)
    L = [1 1]; %Links long.
    
    C2 = (x(1)^2+x(2)^2-L(1)^2-L(2)^2)/(2*prod(L));
    S2 = sqrt(1-C2^2);
q = [atan2(x(2), x(1))-atan2(L(2)*S2, L(1)+L(2)*C2); atan2(S2, C2)];

== matlab function RRmanipulatorsim_/MATLAB Function67 ==
  data: q input; taux output; xdd input
function taux = Mx(q, xdd)
    L = [1 1]; %Links long.
    m = [1 1]; %Links weight.
    
    M = [L(2)*m(2)*(L(2)+cos(q(2))*L(1))+m(1)*L(1)^2+L(1)*m(2)*(L(1)+cos(q(2))*L(2)) L(2)^2*m(2)+L(1)*m(2)*L(2)*cos(q(2));
        L(2)*m(2)*(L(2)+cos(q(2))*L(1)) L(2)^2*m(2)];
    J = [-sin(sum(q))*L(2)-sin(q(1))*L(1) -sin(sum(q))*L(2);
        cos(sum(q))*L(2)+cos(q(1))*L(1) cos(sum(q))*L(2)];
    iJ = J^(-1);
    iJT = (J.')^(-1);
    
    Mx = iJT*M*iJ;
taux = [Mx(1,1)*xdd(1)+Mx(1,2)*xdd(2); Mx(2,1)*xdd(1)+Mx(2,2)*xdd(2)];

% function taux = Mx(q, xdd)
%     M = RRbot.inertia(q');
%     J = RRbot.jacob0(q');
%     J = J(1:N,1:N);
%     iJ = J^(-1);
%     iJT = J.'^(-1);
%     
%     Mx = iJT*M.*iJ;
% taux = [Mx(1,1)*xdd(1)+Mx(1,2)*xdd(2); Mx(2,1)*xdd(1)+Mx(2,2)*xdd(2)];

== matlab function RRmanipulatorsim_/MATLAB Function68 ==
  data: q input; taux output; qd input
function taux = Vx_Fx(q, qd)
    L = [1 1]; %Links long.
    m = [1 1]; %Links weight.
    
    M = [L(2)*m(2)*(L(2)+cos(q(2))*L(1))+m(1)*L(1)^2+L(1)*m(2)*(L(1)+cos(q(2))*L(2)) L(2)^2*m(2)+L(1)*m(2)*L(2)*cos(q(2));
        L(2)*m(2)*(L(2)+cos(q(2))*L(1)) L(2)^2*m(2)];
    V = [-2*m(2)*L(1)*L(2)*sin(q(2))*prod(qd)-m(2)*L(1)*L(2)*sin(q(2))*qd(2)^2;
        m(2)*L(1)*L(2)*sin(q(2))*qd(1)^2];
    G = [0;
        0];
    F = [sign(qd(1));
        sign(qd(2))];
    J = [-sin(sum(q))*L(2)-sin(q(1))*L(1) -sin(sum(q))*L(2);
        cos(sum(q))*L(2)+cos(q(1))*L(1) cos(sum(q))*L(2)];
    iJ = J^(-1);
    iJT = (J')^(-1);
    dJ = [-(sum(qd))*cos(sum(q))*L(2)-qd(1)*cos(q(1))*L(1) -(sum(qd))*cos(sum(q))*L(2);
        -(sum(qd))*sin(sum(q))*L(2)-qd(1)*sin(q(1))*L(1) -(sum(qd))*sin(sum(q))*L(2)];
    
    %dJqd = [dJ(1,1)*qd(1)+dJ(1,2)*qd(2); dJ(2,1)*qd(1)+dJ(2,2)*qd(2)];
    Vx = M*iJ*dJ;
    Vx = V - [Vx(1,1)*qd(1)+Vx(1,2)*qd(2); Vx(2,1)*qd(1)+Vx(2,2)*qd(2)];
    Vx = [iJT(1,1)*Vx(1)+iJT(1,2)*Vx(2); iJT(2,1)*Vx(1)+iJT(2,2)*Vx(2)];
    Gx = [iJT(1,1)*G(1)+iJT(1,2)*G(2); iJT(2,1)*G(1)+iJT(2,2)*G(2)];
    Fx = [iJT(1,1)*F(1)+iJT(1,2)*F(2); iJT(2,1)*F(1)+iJT(2,2)*F(2)];
taux = Vx + Gx + Fx;

% function taux = Vx_Fx(q, qd)
%     C = RRbot.coriolis(q', qd');
%     V = [C(1,1)*qd(1)+C(1,2)*qd(2); C(2,1)*qd(1)+C(2,2)*qd(2)]; %V = Cqd
%     F = -RRbot.friction(qd')';
%     J = RRbot.jacob0(q');
%     J = J(1:N,1:N);
%     iJ = J^(-1);
%     iJT = J.'^(-1);
%     dJ = [-(sum(qd))*cos(sum(q))*LT-qd(1)*cos(q(1))*L1 -(sum(qd))*cos(sum(q))*LT;
%         -(sum(qd))*sin(sum(q))*LT-qd(1)*sin(q(1))*L1 -(sum(qd))*sin(sum(q))*LT];
%     dJqd = [dJ(1,1)*qd(1)+dJ(1,2)*qd(2); dJ(2,1)*qd(1)+dJ(2,2)*qd(2)];
%     
%     Vx = M*iJ;
%     Vx = V - [Vx(1,1)*dJqd(1)+Vx(1,2)*dJqd(2); Vx(2,1)*dJqd(1)+Vx(2,2)*dJqd(2)];
%     Vx = [iJT(1,1)*Vx(1)+iJT(1,2)*Vx(2); iJT(2,1)*Vx(1)+iJT(2,2)*Vx(2)];
%     Fx = [iJT(1,1)*F(1)+iJT(1,2)*F(2); iJT(2,1)*F(1)+iJT(2,2)*F(2)];
% taux = Vx + Fx;

== matlab function RRmanipulatorsim_/MATLAB Function69 ==
  data: q input; x output
function x = kine(q)
    L = [1 1]; %Links long.

x = [cos(sum(q))*L(2)+cos(q(1))*L(1); sin(sum(q))*L(2)+sin(q(1))*L(1)];

== matlab function RRmanipulatorsim_/MATLAB Function70 ==
  data: q input; xd output; qd input
function xd = J(q, qd)
    L = [1 1]; %Links long.

    J = [-sin(sum(q))*L(2)-sin(q(1))*L(1) -sin(sum(q))*L(2);
        cos(sum(q))*L(2)+cos(q(1))*L(1) cos(sum(q))*L(2)];
xd = [J(1,1)*qd(1)+J(1,2)*qd(2); J(2,1)*qd(1)+J(2,2)*qd(2)];

== matlab function RRmanipulatorsim_/MATLAB Function71 ==
  data: q input; tau output; taux input
function tau = JT(q, taux)    
    L = [1 1]; %Links long.

    J = [-sin(sum(q))*L(2)-sin(q(1))*L(1) -sin(sum(q))*L(2);
        cos(sum(q))*L(2)+cos(q(1))*L(1) cos(sum(q))*L(2)];
    JT = J';
tau = [JT(1,1)*taux(1)+JT(1,2)*taux(2); JT(2,1)*taux(1)+JT(2,2)*taux(2)];

% function tau = JT(q, taux)
%     J = RRbot.jacob0(q');
%     JT = J(1:N,1:N)';
% tau = [JT(1,1)*taux(1)+JT(1,2)*taux(2); JT(2,1)*taux(1)+JT(2,2)*taux(2)];

== matlab function RRmanipulatorsim_/MATLAB Function72 ==
  data: x input; q output
function q = ikine(x)
    L = [1 1]; %Links long.
    
    C2 = (x(1)^2+x(2)^2-L(1)^2-L(2)^2)/(2*prod(L));
    S2 = sqrt(1-C2^2);
q = [atan2(x(2), x(1))-atan2(L(2)*S2, L(1)+L(2)*C2); atan2(S2, C2)];

== matlab function RRmanipulatorsim_/MATLAB Function73 ==
  data: q input; x output
function x = kine(q)
    L = [1 1]; %Links long.

x = [cos(sum(q))*L(2)+cos(q(1))*L(1); sin(sum(q))*L(2)+sin(q(1))*L(1)];

== matlab function RRmanipulatorsim_/MATLAB Function6 ==
  data: q input; x output
function x = kine(q)
    L = [1 1]; %Links long.

x = [cos(sum(q))*L(2)+cos(q(1))*L(1); sin(sum(q))*L(2)+sin(q(1))*L(1)];

== matlab function RRmanipulatorsim_/MATLAB Function74 ==
  data: q input; xd output; qd input
function xd = J(q, qd)
    L = [1 1]; %Links long.

    J = [-sin(sum(q))*L(2)-sin(q(1))*L(1) -sin(sum(q))*L(2);
        cos(sum(q))*L(2)+cos(q(1))*L(1) cos(sum(q))*L(2)];
xd = [J(1,1)*qd(1)+J(1,2)*qd(2); J(2,1)*qd(1)+J(2,2)*qd(2)];

== matlab function RRmanipulatorsim_/MATLAB Function75 ==
  data: q input; tau output; taux input
function tau = JT(q, taux)    
    L = [1 1]; %Links long.

    J = [-sin(sum(q))*L(2)-sin(q(1))*L(1) -sin(sum(q))*L(2);
        cos(sum(q))*L(2)+cos(q(1))*L(1) cos(sum(q))*L(2)];
    JT = J';
tau = [JT(1,1)*taux(1)+JT(1,2)*taux(2); JT(2,1)*taux(1)+JT(2,2)*taux(2)];

% function tau = JT(q, taux)
%     J = RRbot.jacob0(q');
%     JT = J(1:N,1:N)';
% tau = [JT(1,1)*taux(1)+JT(1,2)*taux(2); JT(2,1)*taux(1)+JT(2,2)*taux(2)];

== matlab function RRmanipulatorsim_/MATLAB Function76 ==
  data: x input; q output
function q = ikine(x)
    L = [1 1]; %Links long.
    
    C2 = (x(1)^2+x(2)^2-L(1)^2-L(2)^2)/(2*prod(L));
    S2 = sqrt(1-C2^2);
q = [atan2(x(2), x(1))-atan2(L(2)*S2, L(1)+L(2)*C2); atan2(S2, C2)];

== matlab function RRmanipulatorsim_/MATLAB Function77 ==
  data: q input; taux output; xdd input
function taux = Mx(q, xdd)
    L = [1 1]; %Links long.
    m = [1 1]; %Links weight.
    
    M = [L(2)*m(2)*(L(2)+cos(q(2))*L(1))+m(1)*L(1)^2+L(1)*m(2)*(L(1)+cos(q(2))*L(2)) L(2)^2*m(2)+L(1)*m(2)*L(2)*cos(q(2));
        L(2)*m(2)*(L(2)+cos(q(2))*L(1)) L(2)^2*m(2)];
    J = [-sin(sum(q))*L(2)-sin(q(1))*L(1) -sin(sum(q))*L(2);
        cos(sum(q))*L(2)+cos(q(1))*L(1) cos(sum(q))*L(2)];
    iJ = J^(-1);
    iJT = (J.')^(-1);
    
    Mx = iJT*M*iJ;
taux = [Mx(1,1)*xdd(1)+Mx(1,2)*xdd(2); Mx(2,1)*xdd(1)+Mx(2,2)*xdd(2)];

% function taux = Mx(q, xdd)
%     M = RRbot.inertia(q');
%     J = RRbot.jacob0(q');
%     J = J(1:N,1:N);
%     iJ = J^(-1);
%     iJT = J.'^(-1);
%     
%     Mx = iJT*M.*iJ;
% taux = [Mx(1,1)*xdd(1)+Mx(1,2)*xdd(2); Mx(2,1)*xdd(1)+Mx(2,2)*xdd(2)];

== matlab function RRmanipulatorsim_/MATLAB Function78 ==
  data: q input; taux output; qd input
function taux = Vx_Fx(q, qd)
    L = [1 1]; %Links long.
    m = [1 1]; %Links weight.
    
    M = [L(2)*m(2)*(L(2)+cos(q(2))*L(1))+m(1)*L(1)^2+L(1)*m(2)*(L(1)+cos(q(2))*L(2)) L(2)^2*m(2)+L(1)*m(2)*L(2)*cos(q(2));
        L(2)*m(2)*(L(2)+cos(q(2))*L(1)) L(2)^2*m(2)];
    V = [-2*m(2)*L(1)*L(2)*sin(q(2))*prod(qd)-m(2)*L(1)*L(2)*sin(q(2))*qd(2)^2;
        m(2)*L(1)*L(2)*sin(q(2))*qd(1)^2];
    G = [0;
        0];
    F = [sign(qd(1));
        sign(qd(2))];
    J = [-sin(sum(q))*L(2)-sin(q(1))*L(1) -sin(sum(q))*L(2);
        cos(sum(q))*L(2)+cos(q(1))*L(1) cos(sum(q))*L(2)];
    iJ = J^(-1);
    iJT = (J')^(-1);
    dJ = [-(sum(qd))*cos(sum(q))*L(2)-qd(1)*cos(q(1))*L(1) -(sum(qd))*cos(sum(q))*L(2);
        -(sum(qd))*sin(sum(q))*L(2)-qd(1)*sin(q(1))*L(1) -(sum(qd))*sin(sum(q))*L(2)];
    
    %dJqd = [dJ(1,1)*qd(1)+dJ(1,2)*qd(2); dJ(2,1)*qd(1)+dJ(2,2)*qd(2)];
    Vx = M*iJ*dJ;
    Vx = V - [Vx(1,1)*qd(1)+Vx(1,2)*qd(2); Vx(2,1)*qd(1)+Vx(2,2)*qd(2)];
    Vx = [iJT(1,1)*Vx(1)+iJT(1,2)*Vx(2); iJT(2,1)*Vx(1)+iJT(2,2)*Vx(2)];
    Gx = [iJT(1,1)*G(1)+iJT(1,2)*G(2); iJT(2,1)*G(1)+iJT(2,2)*G(2)];
    Fx = [iJT(1,1)*F(1)+iJT(1,2)*F(2); iJT(2,1)*F(1)+iJT(2,2)*F(2)];
taux = Vx + Gx + Fx;

% function taux = Vx_Fx(q, qd)
%     C = RRbot.coriolis(q', qd');
%     V = [C(1,1)*qd(1)+C(1,2)*qd(2); C(2,1)*qd(1)+C(2,2)*qd(2)]; %V = Cqd
%     F = -RRbot.friction(qd')';
%     J = RRbot.jacob0(q');
%     J = J(1:N,1:N);
%     iJ = J^(-1);
%     iJT = J.'^(-1);
%     dJ = [-(sum(qd))*cos(sum(q))*LT-qd(1)*cos(q(1))*L1 -(sum(qd))*cos(sum(q))*LT;
%         -(sum(qd))*sin(sum(q))*LT-qd(1)*sin(q(1))*L1 -(sum(qd))*sin(sum(q))*LT];
%     dJqd = [dJ(1,1)*qd(1)+dJ(1,2)*qd(2); dJ(2,1)*qd(1)+dJ(2,2)*qd(2)];
%     
%     Vx = M*iJ;
%     Vx = V - [Vx(1,1)*dJqd(1)+Vx(1,2)*dJqd(2); Vx(2,1)*dJqd(1)+Vx(2,2)*dJqd(2)];
%     Vx = [iJT(1,1)*Vx(1)+iJT(1,2)*Vx(2); iJT(2,1)*Vx(1)+iJT(2,2)*Vx(2)];
%     Fx = [iJT(1,1)*F(1)+iJT(1,2)*F(2); iJT(2,1)*F(1)+iJT(2,2)*F(2)];
% taux = Vx + Fx;

== matlab function RRmanipulatorsim_/MATLAB Function79 ==
  data: q input; x output
function x = kine(q)
    L = [1 1]; %Links long.

x = [cos(sum(q))*L(2)+cos(q(1))*L(1); sin(sum(q))*L(2)+sin(q(1))*L(1)];

== matlab function RRmanipulatorsim_/MATLAB Function80 ==
  data: q input; xd output; qd input
function xd = J(q, qd)
    L = [1 1]; %Links long.

    J = [-sin(sum(q))*L(2)-sin(q(1))*L(1) -sin(sum(q))*L(2);
        cos(sum(q))*L(2)+cos(q(1))*L(1) cos(sum(q))*L(2)];
xd = [J(1,1)*qd(1)+J(1,2)*qd(2); J(2,1)*qd(1)+J(2,2)*qd(2)];

== matlab function RRmanipulatorsim_/MATLAB Function81 ==
  data: q input; tau output; taux input
function tau = JT(q, taux)    
    L = [1 1]; %Links long.

    J = [-sin(sum(q))*L(2)-sin(q(1))*L(1) -sin(sum(q))*L(2);
        cos(sum(q))*L(2)+cos(q(1))*L(1) cos(sum(q))*L(2)];
    JT = J';
tau = [JT(1,1)*taux(1)+JT(1,2)*taux(2); JT(2,1)*taux(1)+JT(2,2)*taux(2)];

% function tau = JT(q, taux)
%     J = RRbot.jacob0(q');
%     JT = J(1:N,1:N)';
% tau = [JT(1,1)*taux(1)+JT(1,2)*taux(2); JT(2,1)*taux(1)+JT(2,2)*taux(2)];

== matlab function RRmanipulatorsim_/MATLAB Function82 ==
  data: x input; q output
function q = ikine(x)
    L = [1 1]; %Links long.
    
    C2 = (x(1)^2+x(2)^2-L(1)^2-L(2)^2)/(2*prod(L));
    S2 = sqrt(1-C2^2);
q = [atan2(x(2), x(1))-atan2(L(2)*S2, L(1)+L(2)*C2); atan2(S2, C2)];

== matlab function RRmanipulatorsim_/MATLAB Function7 ==
  data: q input; xd output; qd input
function xd = J(q, qd)
    L = [1 1]; %Links long.

    J = [-sin(sum(q))*L(2)-sin(q(1))*L(1) -sin(sum(q))*L(2);
        cos(sum(q))*L(2)+cos(q(1))*L(1) cos(sum(q))*L(2)];
xd = [J(1,1)*qd(1)+J(1,2)*qd(2); J(2,1)*qd(1)+J(2,2)*qd(2)];

== matlab function RRmanipulatorsim_/MATLAB Function83 ==
  data: q input; taux output; xdd input
function taux = Mx(q, xdd)
    L = [1 1]; %Links long.
    m = [1 1]; %Links weight.
    
    M = [L(2)*m(2)*(L(2)+cos(q(2))*L(1))+m(1)*L(1)^2+L(1)*m(2)*(L(1)+cos(q(2))*L(2)) L(2)^2*m(2)+L(1)*m(2)*L(2)*cos(q(2));
        L(2)*m(2)*(L(2)+cos(q(2))*L(1)) L(2)^2*m(2)];
    J = [-sin(sum(q))*L(2)-sin(q(1))*L(1) -sin(sum(q))*L(2);
        cos(sum(q))*L(2)+cos(q(1))*L(1) cos(sum(q))*L(2)];
    iJ = J^(-1);
    iJT = (J.')^(-1);
    
    Mx = iJT*M*iJ;
taux = [Mx(1,1)*xdd(1)+Mx(1,2)*xdd(2); Mx(2,1)*xdd(1)+Mx(2,2)*xdd(2)];

% function taux = Mx(q, xdd)
%     M = RRbot.inertia(q');
%     J = RRbot.jacob0(q');
%     J = J(1:N,1:N);
%     iJ = J^(-1);
%     iJT = J.'^(-1);
%     
%     Mx = iJT*M.*iJ;
% taux = [Mx(1,1)*xdd(1)+Mx(1,2)*xdd(2); Mx(2,1)*xdd(1)+Mx(2,2)*xdd(2)];

== matlab function RRmanipulatorsim_/MATLAB Function84 ==
  data: q input; taux output; qd input
function taux = Vx_Fx(q, qd)
    L = [1 1]; %Links long.
    m = [1 1]; %Links weight.
    
    M = [L(2)*m(2)*(L(2)+cos(q(2))*L(1))+m(1)*L(1)^2+L(1)*m(2)*(L(1)+cos(q(2))*L(2)) L(2)^2*m(2)+L(1)*m(2)*L(2)*cos(q(2));
        L(2)*m(2)*(L(2)+cos(q(2))*L(1)) L(2)^2*m(2)];
    V = [-2*m(2)*L(1)*L(2)*sin(q(2))*prod(qd)-m(2)*L(1)*L(2)*sin(q(2))*qd(2)^2;
        m(2)*L(1)*L(2)*sin(q(2))*qd(1)^2];
    G = [0;
        0];
    F = [sign(qd(1));
        sign(qd(2))];
    J = [-sin(sum(q))*L(2)-sin(q(1))*L(1) -sin(sum(q))*L(2);
        cos(sum(q))*L(2)+cos(q(1))*L(1) cos(sum(q))*L(2)];
    iJ = J^(-1);
    iJT = (J')^(-1);
    dJ = [-(sum(qd))*cos(sum(q))*L(2)-qd(1)*cos(q(1))*L(1) -(sum(qd))*cos(sum(q))*L(2);
        -(sum(qd))*sin(sum(q))*L(2)-qd(1)*sin(q(1))*L(1) -(sum(qd))*sin(sum(q))*L(2)];
    
    %dJqd = [dJ(1,1)*qd(1)+dJ(1,2)*qd(2); dJ(2,1)*qd(1)+dJ(2,2)*qd(2)];
    Vx = M*iJ*dJ;
    Vx = V - [Vx(1,1)*qd(1)+Vx(1,2)*qd(2); Vx(2,1)*qd(1)+Vx(2,2)*qd(2)];
    Vx = [iJT(1,1)*Vx(1)+iJT(1,2)*Vx(2); iJT(2,1)*Vx(1)+iJT(2,2)*Vx(2)];
    Gx = [iJT(1,1)*G(1)+iJT(1,2)*G(2); iJT(2,1)*G(1)+iJT(2,2)*G(2)];
    Fx = [iJT(1,1)*F(1)+iJT(1,2)*F(2); iJT(2,1)*F(1)+iJT(2,2)*F(2)];
taux = Vx + Gx + Fx;

% function taux = Vx_Fx(q, qd)
%     C = RRbot.coriolis(q', qd');
%     V = [C(1,1)*qd(1)+C(1,2)*qd(2); C(2,1)*qd(1)+C(2,2)*qd(2)]; %V = Cqd
%     F = -RRbot.friction(qd')';
%     J = RRbot.jacob0(q');
%     J = J(1:N,1:N);
%     iJ = J^(-1);
%     iJT = J.'^(-1);
%     dJ = [-(sum(qd))*cos(sum(q))*LT-qd(1)*cos(q(1))*L1 -(sum(qd))*cos(sum(q))*LT;
%         -(sum(qd))*sin(sum(q))*LT-qd(1)*sin(q(1))*L1 -(sum(qd))*sin(sum(q))*LT];
%     dJqd = [dJ(1,1)*qd(1)+dJ(1,2)*qd(2); dJ(2,1)*qd(1)+dJ(2,2)*qd(2)];
%     
%     Vx = M*iJ;
%     Vx = V - [Vx(1,1)*dJqd(1)+Vx(1,2)*dJqd(2); Vx(2,1)*dJqd(1)+Vx(2,2)*dJqd(2)];
%     Vx = [iJT(1,1)*Vx(1)+iJT(1,2)*Vx(2); iJT(2,1)*Vx(1)+iJT(2,2)*Vx(2)];
%     Fx = [iJT(1,1)*F(1)+iJT(1,2)*F(2); iJT(2,1)*F(1)+iJT(2,2)*F(2)];
% taux = Vx + Fx;

== matlab function RRmanipulatorsim_/MATLAB Function85 ==
  data: q input; x output
function x = kine(q)
    L = [1 1]; %Links long.

x = [cos(sum(q))*L(2)+cos(q(1))*L(1); sin(sum(q))*L(2)+sin(q(1))*L(1)];

== matlab function RRmanipulatorsim_/MATLAB Function86 ==
  data: q input; xd output; qd input
function xd = J(q, qd)
    L = [1 1]; %Links long.

    J = [-sin(sum(q))*L(2)-sin(q(1))*L(1) -sin(sum(q))*L(2);
        cos(sum(q))*L(2)+cos(q(1))*L(1) cos(sum(q))*L(2)];
xd = [J(1,1)*qd(1)+J(1,2)*qd(2); J(2,1)*qd(1)+J(2,2)*qd(2)];

== matlab function RRmanipulatorsim_/MATLAB Function87 ==
  data: q input; tau output; taux input
function tau = JT(q, taux)    
    L = [1 1]; %Links long.

    J = [-sin(sum(q))*L(2)-sin(q(1))*L(1) -sin(sum(q))*L(2);
        cos(sum(q))*L(2)+cos(q(1))*L(1) cos(sum(q))*L(2)];
    JT = J';
tau = [JT(1,1)*taux(1)+JT(1,2)*taux(2); JT(2,1)*taux(1)+JT(2,2)*taux(2)];

% function tau = JT(q, taux)
%     J = RRbot.jacob0(q');
%     JT = J(1:N,1:N)';
% tau = [JT(1,1)*taux(1)+JT(1,2)*taux(2); JT(2,1)*taux(1)+JT(2,2)*taux(2)];

== matlab function RRmanipulatorsim_/MATLAB Function88 ==
  data: x input; q output
function q = ikine(x)
    L = [1 1]; %Links long.
    
    C2 = (x(1)^2+x(2)^2-L(1)^2-L(2)^2)/(2*prod(L));
    S2 = sqrt(1-C2^2);
q = [atan2(x(2), x(1))-atan2(L(2)*S2, L(1)+L(2)*C2); atan2(S2, C2)];

== matlab function RRmanipulatorsim_/MATLAB Function89 ==
  data: q input; taux output; xdd input
function taux = Mx(q, xdd)
    L = [1 1]; %Links long.
    m = [1 1]; %Links weight.
    
    M = [L(2)*m(2)*(L(2)+cos(q(2))*L(1))+m(1)*L(1)^2+L(1)*m(2)*(L(1)+cos(q(2))*L(2)) L(2)^2*m(2)+L(1)*m(2)*L(2)*cos(q(2));
        L(2)*m(2)*(L(2)+cos(q(2))*L(1)) L(2)^2*m(2)];
    J = [-sin(sum(q))*L(2)-sin(q(1))*L(1) -sin(sum(q))*L(2);
        cos(sum(q))*L(2)+cos(q(1))*L(1) cos(sum(q))*L(2)];
    iJ = J^(-1);
    iJT = (J.')^(-1);
    
    Mx = iJT*M*iJ;
taux = [Mx(1,1)*xdd(1)+Mx(1,2)*xdd(2); Mx(2,1)*xdd(1)+Mx(2,2)*xdd(2)];

% function taux = Mx(q, xdd)
%     M = RRbot.inertia(q');
%     J = RRbot.jacob0(q');
%     J = J(1:N,1:N);
%     iJ = J^(-1);
%     iJT = J.'^(-1);
%     
%     Mx = iJT*M.*iJ;
% taux = [Mx(1,1)*xdd(1)+Mx(1,2)*xdd(2); Mx(2,1)*xdd(1)+Mx(2,2)*xdd(2)];

== matlab function RRmanipulatorsim_/MATLAB Function90 ==
  data: q input; taux output; qd input
function taux = Vx_Fx(q, qd)
    L = [1 1]; %Links long.
    m = [1 1]; %Links weight.
    
    M = [L(2)*m(2)*(L(2)+cos(q(2))*L(1))+m(1)*L(1)^2+L(1)*m(2)*(L(1)+cos(q(2))*L(2)) L(2)^2*m(2)+L(1)*m(2)*L(2)*cos(q(2));
        L(2)*m(2)*(L(2)+cos(q(2))*L(1)) L(2)^2*m(2)];
    V = [-2*m(2)*L(1)*L(2)*sin(q(2))*prod(qd)-m(2)*L(1)*L(2)*sin(q(2))*qd(2)^2;
        m(2)*L(1)*L(2)*sin(q(2))*qd(1)^2];
    G = [0;
        0];
    F = [sign(qd(1));
        sign(qd(2))];
    J = [-sin(sum(q))*L(2)-sin(q(1))*L(1) -sin(sum(q))*L(2);
        cos(sum(q))*L(2)+cos(q(1))*L(1) cos(sum(q))*L(2)];
    iJ = J^(-1);
    iJT = (J')^(-1);
    dJ = [-(sum(qd))*cos(sum(q))*L(2)-qd(1)*cos(q(1))*L(1) -(sum(qd))*cos(sum(q))*L(2);
        -(sum(qd))*sin(sum(q))*L(2)-qd(1)*sin(q(1))*L(1) -(sum(qd))*sin(sum(q))*L(2)];
    
    %dJqd = [dJ(1,1)*qd(1)+dJ(1,2)*qd(2); dJ(2,1)*qd(1)+dJ(2,2)*qd(2)];
    Vx = M*iJ*dJ;
    Vx = V - [Vx(1,1)*qd(1)+Vx(1,2)*qd(2); Vx(2,1)*qd(1)+Vx(2,2)*qd(2)];
    Vx = [iJT(1,1)*Vx(1)+iJT(1,2)*Vx(2); iJT(2,1)*Vx(1)+iJT(2,2)*Vx(2)];
    Gx = [iJT(1,1)*G(1)+iJT(1,2)*G(2); iJT(2,1)*G(1)+iJT(2,2)*G(2)];
    Fx = [iJT(1,1)*F(1)+iJT(1,2)*F(2); iJT(2,1)*F(1)+iJT(2,2)*F(2)];
taux = Vx + Gx + Fx;

% function taux = Vx_Fx(q, qd)
%     C = RRbot.coriolis(q', qd');
%     V = [C(1,1)*qd(1)+C(1,2)*qd(2); C(2,1)*qd(1)+C(2,2)*qd(2)]; %V = Cqd
%     F = -RRbot.friction(qd')';
%     J = RRbot.jacob0(q');
%     J = J(1:N,1:N);
%     iJ = J^(-1);
%     iJT = J.'^(-1);
%     dJ = [-(sum(qd))*cos(sum(q))*LT-qd(1)*cos(q(1))*L1 -(sum(qd))*cos(sum(q))*LT;
%         -(sum(qd))*sin(sum(q))*LT-qd(1)*sin(q(1))*L1 -(sum(qd))*sin(sum(q))*LT];
%     dJqd = [dJ(1,1)*qd(1)+dJ(1,2)*qd(2); dJ(2,1)*qd(1)+dJ(2,2)*qd(2)];
%     
%     Vx = M*iJ;
%     Vx = V - [Vx(1,1)*dJqd(1)+Vx(1,2)*dJqd(2); Vx(2,1)*dJqd(1)+Vx(2,2)*dJqd(2)];
%     Vx = [iJT(1,1)*Vx(1)+iJT(1,2)*Vx(2); iJT(2,1)*Vx(1)+iJT(2,2)*Vx(2)];
%     Fx = [iJT(1,1)*F(1)+iJT(1,2)*F(2); iJT(2,1)*F(1)+iJT(2,2)*F(2)];
% taux = Vx + Fx;

== matlab function RRmanipulatorsim_/MATLAB Function91 ==
  data: q input; x output
function x = kine(q)
    L = [1 1]; %Links long.

x = [cos(sum(q))*L(2)+cos(q(1))*L(1); sin(sum(q))*L(2)+sin(q(1))*L(1)];

== matlab function RRmanipulatorsim_/MATLAB Function92 ==
  data: q input; xd output; qd input
function xd = J(q, qd)
    L = [1 1]; %Links long.

    J = [-sin(sum(q))*L(2)-sin(q(1))*L(1) -sin(sum(q))*L(2);
        cos(sum(q))*L(2)+cos(q(1))*L(1) cos(sum(q))*L(2)];
xd = [J(1,1)*qd(1)+J(1,2)*qd(2); J(2,1)*qd(1)+J(2,2)*qd(2)];

== matlab function RRmanipulatorsim_/MATLAB Function93 ==
  data: q input; tau output; taux input
function tau = JT(q, taux)    
    L = [1 1]; %Links long.

    J = [-sin(sum(q))*L(2)-sin(q(1))*L(1) -sin(sum(q))*L(2);
        cos(sum(q))*L(2)+cos(q(1))*L(1) cos(sum(q))*L(2)];
    JT = J';
tau = [JT(1,1)*taux(1)+JT(1,2)*taux(2); JT(2,1)*taux(1)+JT(2,2)*taux(2)];

% function tau = JT(q, taux)
%     J = RRbot.jacob0(q');
%     JT = J(1:N,1:N)';
% tau = [JT(1,1)*taux(1)+JT(1,2)*taux(2); JT(2,1)*taux(1)+JT(2,2)*taux(2)];

== matlab function RRmanipulatorsim_/MATLAB Function8 ==
  data: q input; tau output; taux input
function tau = JT(q, taux)    
    L = [1 1]; %Links long.

    J = [-sin(sum(q))*L(2)-sin(q(1))*L(1) -sin(sum(q))*L(2);
        cos(sum(q))*L(2)+cos(q(1))*L(1) cos(sum(q))*L(2)];
    JT = J';
tau = [JT(1,1)*taux(1)+JT(1,2)*taux(2); JT(2,1)*taux(1)+JT(2,2)*taux(2)];

% function tau = JT(q, taux)
%     J = RRbot.jacob0(q');
%     JT = J(1:N,1:N)';
% tau = [JT(1,1)*taux(1)+JT(1,2)*taux(2); JT(2,1)*taux(1)+JT(2,2)*taux(2)];

== matlab function RRmanipulatorsim_/MATLAB Function94 ==
  data: x input; q output
function q = ikine(x)
    L = [1 1]; %Links long.
    
    C2 = (x(1)^2+x(2)^2-L(1)^2-L(2)^2)/(2*prod(L));
    S2 = sqrt(1-C2^2);
q = [atan2(x(2), x(1))-atan2(L(2)*S2, L(1)+L(2)*C2); atan2(S2, C2)];

== matlab function RRmanipulatorsim_/MATLAB Function100 ==
  data: x input; q output
function q = ikine(x)
    L = [1 1]; %Links long.
    
    C2 = (x(1)^2+x(2)^2-L(1)^2-L(2)^2)/(2*prod(L));
    S2 = sqrt(1-C2^2);
q = [atan2(x(2), x(1))-atan2(L(2)*S2, L(1)+L(2)*C2); atan2(S2, C2)];

== matlab function RRmanipulatorsim_/MATLAB Function101 ==
  data: q input; taux output; xdd input
function taux = Mx(q, xdd)
    L = [1 1]; %Links long.
    m = [1 1]; %Links weight.
    
    M = [L(2)*m(2)*(L(2)+cos(q(2))*L(1))+m(1)*L(1)^2+L(1)*m(2)*(L(1)+cos(q(2))*L(2)) L(2)^2*m(2)+L(1)*m(2)*L(2)*cos(q(2));
        L(2)*m(2)*(L(2)+cos(q(2))*L(1)) L(2)^2*m(2)];
    J = [-sin(sum(q))*L(2)-sin(q(1))*L(1) -sin(sum(q))*L(2);
        cos(sum(q))*L(2)+cos(q(1))*L(1) cos(sum(q))*L(2)];
    iJ = J^(-1);
    iJT = (J.')^(-1);
    
    Mx = iJT*M*iJ;
taux = [Mx(1,1)*xdd(1)+Mx(1,2)*xdd(2); Mx(2,1)*xdd(1)+Mx(2,2)*xdd(2)];

% function taux = Mx(q, xdd)
%     M = RRbot.inertia(q');
%     J = RRbot.jacob0(q');
%     J = J(1:N,1:N);
%     iJ = J^(-1);
%     iJT = J.'^(-1);
%     
%     Mx = iJT*M.*iJ;
% taux = [Mx(1,1)*xdd(1)+Mx(1,2)*xdd(2); Mx(2,1)*xdd(1)+Mx(2,2)*xdd(2)];
